simulink model "test_shading_control"  (Simulink 8.2)
settings: Solver=ode45  StartTime=180*24*3600  StopTime=190*24*3600  RelTol=1e-3
libraries: carnot x3, simulink x1
settings Model: Creator=drhf  LastModifiedBy=drhf

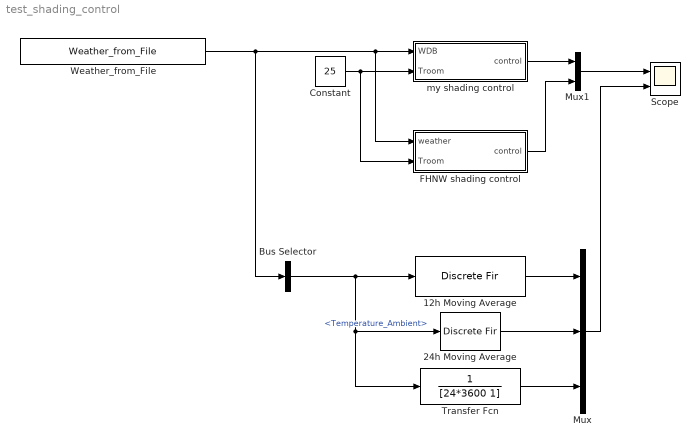
== system test_shading_control ==
  12h Moving Average : DiscreteFir  Coefficients=ones(1,24)*(1/24)  SampleTime=1800  AccumDataTypeStr=Inherit: Same as product output  RndMeth=Nearest
  24h Moving Average : DiscreteFir  Coefficients=ones(1,24)*(1/24)  SampleTime=60  AccumDataTypeStr=Inherit: Same as product output  RndMeth=Nearest
  Bus Selector : BusSelector  OutputSignals=Temperature_Ambient
  Constant : Constant  Value=25
  FHNW shading control : Subsystem
  Mux : Mux  Inputs=3
  Mux1 : Mux  Inputs=2
  Scope : Scope  NumInputPorts=2
      settings: TickLabels=on  YMin=-7.5~0  YMax=35~0.0019  SampleTime=3600*3
  Transfer Fcn : TransferFcn  Denominator=[24*3600 1]
  Weather_from_File : carnot/Weather/Weather_from_File  file=DE_TRY2010_12_averageYear  ext=.mat
  my shading control : Subsystem
  wires:
  Bus Selector/1 -> 12h Moving Average/1, Transfer Fcn/1, 24h Moving Average/1  "<Temperature_Ambient>"
  Weather_from_File/1 -> Bus Selector/1, my shading control/1(WDB), FHNW shading control/1(weather)
  Constant/1 -> my shading control/2(Troom), FHNW shading control/2(Troom)
  12h Moving Average/1 -> Mux/1
  Transfer Fcn/1 -> Mux/3
  Mux/1 -> Scope/2
  my shading control/1(control) -> Mux1/1
  FHNW shading control/1(control) -> Mux1/2
  Mux1/1 -> Scope/1
  24h Moving Average/1 -> Mux/2

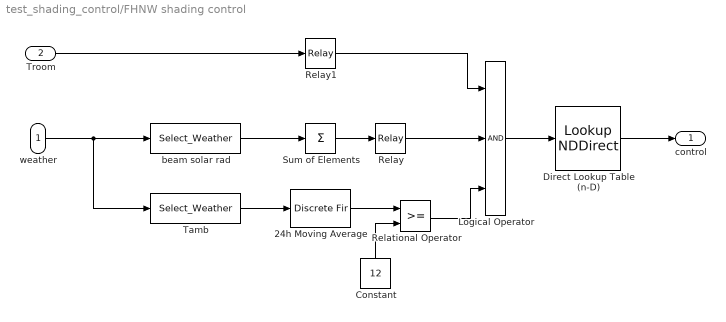
== system test_shading_control/FHNW shading control ==
  weather : Inport
  Troom : Inport  Port=2
  24h Moving Average : DiscreteFir  Coefficients=ones(1,24)*(1/24)  SampleTime=60  AccumDataTypeStr=Inherit: Same as product output  RndMeth=Nearest
  Constant : Constant  Value=12
  Direct Lookup Table (n-D) : LookupNDDirect  NumberOfTableDimensions=1  Table=[1 1-0.75]
  Logical Operator : Logic  Inputs=3  AllPortsSameDT=off  OutDataTypeStr=boolean
  Relational Operator : RelationalOperator  OutDataTypeStr=boolean
  Relay : Relay  OnSwitchValue=300  OffSwitchValue=200
  Relay1 : Relay  OnSwitchValue=23.8  OffSwitchValue=22.8
  Sum of Elements : Sum  Inputs=+
  Tamb : carnot/Weather/Select_Weather  SystemSampleTime=-1  v=6
  beam solar rad : carnot/Weather/Select_Weather  SystemSampleTime=-1  v=[17 18]
  control : Outport
  wires:
  beam solar rad/1 -> Sum of Elements/1
  24h Moving Average/1 -> Relational Operator/1
  Logical Operator/1 -> Direct Lookup Table (n-D)/1
  Sum of Elements/1 -> Relay/1
  Relay/1 -> Logical Operator/2
  Relational Operator/1 -> Logical Operator/3
  Troom/1 -> Relay1/1
  Direct Lookup Table (n-D)/1 -> control/1
  weather/1 -> Tamb/1, beam solar rad/1
  Relay1/1 -> Logical Operator/1
  Constant/1 -> Relational Operator/2
  Tamb/1 -> 24h Moving Average/1

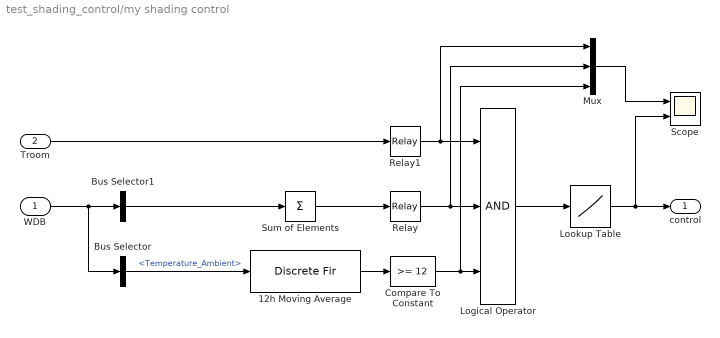
== system test_shading_control/my shading control ==
  WDB : Inport
  Troom : Inport  Port=2
  12h Moving Average : DiscreteFir  Coefficients=ones(1,24)*(1/24)  SampleTime=1800  AccumDataTypeStr=Inherit: Same as product output  RndMeth=Nearest
  Bus Selector : BusSelector  OutputSignals=Temperature_Ambient
  Bus Selector1 : BusSelector  OutputSignals=Solar_Radiation_direct_surface,Solar_Radiation_diffuse_surface  OutputAsBus=on
  Compare To Constant : simulink/Logic and Bit Operations/Compare To Constant  SystemSampleTime=-1  relop=>=  const=12  LogicOutDataTypeMode=uint8
  Logical Operator : Logic  Inputs=3  AllPortsSameDT=off  OutDataTypeStr=boolean
  Lookup Table : Lookup  InputValues=[0 1]  Table=[1 1-0.75]  OutDataTypeStr=double
  Mux : Mux  Inputs=3
  Relay : Relay  OnSwitchValue=300  OffSwitchValue=200  OutDataTypeStr=uint8
  Relay1 : Relay  OnSwitchValue=23.8  OffSwitchValue=22.8  OutDataTypeStr=uint8
  Scope : Scope  NumInputPorts=2
      settings: TickLabels=on  YMin=-7.5~0  YMax=35~0.0019  SampleTime=3600*3
  Sum of Elements : Sum  Inputs=+
  control : Outport
  wires:
  Bus Selector1/1 -> Sum of Elements/1
  12h Moving Average/1 -> Compare To Constant/1
  Logical Operator/1 -> Lookup Table/1
  Sum of Elements/1 -> Relay/1
  Relay/1 -> Logical Operator/2, Mux/2
  Compare To Constant/1 -> Logical Operator/3, Mux/3
  Troom/1 -> Relay1/1
  Lookup Table/1 -> control/1, Scope/2
  WDB/1 -> Bus Selector1/1, Bus Selector/1
  Relay1/1 -> Logical Operator/1, Mux/1
  Bus Selector/1 -> 12h Moving Average/1  "<Temperature_Ambient>"
  Mux/1 -> Scope/1
